simulink model "HeatShield_ID_Test"  (R2019a)
settings: Solver=VariableStepAuto  StartTime=0.0  StopTime=16000  RelTol=1e-3
model workspace (MAT data in the model file):
  MCOS : class17 (value not decoded)
  resultIDSimulink = [0 2 4 6 8 10 12 14 16 18 20 22 ... (24300 elements, 8100x3)]
undefined symbols (not defined in the file): model
libraries: slident x1, HeatLibrary x1
(part 2 of 2)

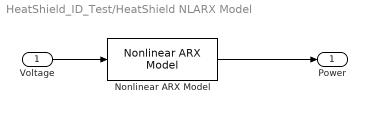
== system HeatShield_ID_Test/HeatShield NLARX Model ==
  Voltage : Inport
  Nonlinear ARX Model : slident/Models/Nonlinear ARX Model  sys=HeatShield_model1  ICspec=Input and output values  X0=0  U0=25  Y0=31
      settings: SourceProductName=System Identification Toolbox  SourceProductBaseCode=ID
  Power : Outport
  wires:
  Voltage/1 -> Nonlinear ARX Model/1
  Nonlinear ARX Model/1 -> Power/1
